simulink model "DC_Motor_BrakeMode_Simplified"  (R2018a)
settings: Solver=VariableStepAuto  StartTime=0.0  StopTime=10.0  FixedStep=1e-5  RelTol=1e-3
settings Model: Creator=Thomas  LastModifiedBy=Thomas

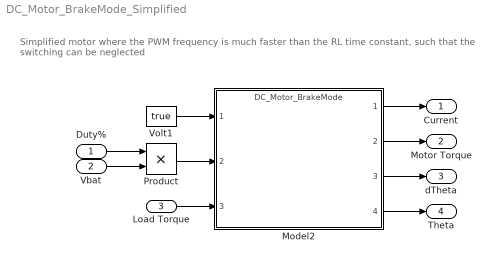
== system DC_Motor_BrakeMode_Simplified ==
  note: Simplified motor where the PWM frequency is much faster than the RL time constant, such that the switching can be neglected
  Duty% : Inport  OutDataTypeStr=double
  Vbat : Inport  Port=2  OutDataTypeStr=double
  Load Torque : Inport  Port=3  OutDataTypeStr=double
  Model2 : ModelReference  ModelNameDialog=DC_Motor_BrakeMode  SimulationMode=Normal  ModelReferenceVersion=1.16
  Product : Product
  Volt1 : Constant  Value=true
  Current : Outport
  Motor Torque : Outport  Port=2
  dTheta : Outport  Port=3
  Theta : Outport  Port=4
  wires:
  Product/1 -> Model2/2
  Volt1/1 -> Model2/1
  Load Torque/1 -> Model2/3
  Model2/4 -> Theta/1
  Model2/3 -> dTheta/1
  Model2/2 -> Motor Torque/1
  Model2/1 -> Current/1
  Vbat/1 -> Product/2
  Duty%/1 -> Product/1
